simulink model "CubeX_LQR_2D"  (R2016b)
settings: Solver=FixedStepDiscrete  StartTime=0.0  StopTime=inf  FixedStep=Ts.base  RelTol=1e-3
PreLoadFcn:
  | waijung.modelPreload; % Required for working with Waijung Blockset. Do not remove.
InitFcn:
  | cubeparameters
  | LQR_2d
undefined symbols (not defined in the file): CPHA_1Edge, CPOL_Low, deg_, Duplex, FirstBit_MSB, Full, g, imu, K_lqr, Link, LQFP100, ST, STM32F407VG, STM32F4DISCOVERY, Ts
libraries: simulink x58, stm32f4_i2c_lib x12, stm32f4_io_lib x6, cube_lib x4, stm32f4_spi_lib x4, stm32f4_adc_lib x1, stm32f4_device_config_lib x1, BC_USB x1
(part 3 of 4)

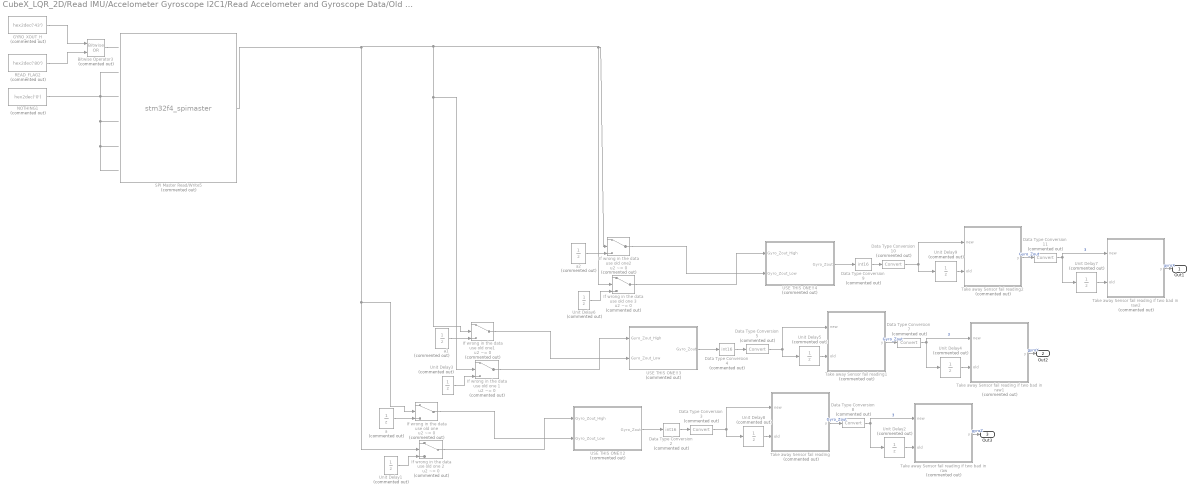
== system CubeX_LQR_2D/Read IMU/Accelometer Gyroscope I2C1/Read Accelometer and Gyroscope Data/Old gyro get data Used during SPI before ==
  " a" : UnitDelay  Commented=on  SampleTime=-1
  " a1" : UnitDelay  Commented=on  SampleTime=-1
  " a2" : UnitDelay  Commented=on  SampleTime=-1
  Bitwise Operator3 : simulink/Logic and Bit Operations/Bitwise Operator  Commented=on  logicop=OR  UseBitMask=off  NumInputPorts=2  BitMask=bin2dec('11011001')  BitMaskRealWorld=Stored Integer
  Data Type Conversion{3,5,7..8,10..11} (6 alike) : DataTypeConversion  Commented=on
  Data Type Conversion2 : DataTypeConversion  Commented=on  OutDataTypeStr=int16
  Data Type Conversion4 : DataTypeConversion  Commented=on  OutDataTypeStr=int16
  Data Type Conversion9 : DataTypeConversion  Commented=on  OutDataTypeStr=int16
  GYRO_XOUT_H : Constant  Commented=on  Value=hex2dec('43')  OutDataTypeStr=uint8
  If wrong in the data use old one : Switch  Commented=on  Criteria=u2 ~= 0
  If wrong in the data use old one 1 : Switch  Commented=on  Criteria=u2 ~= 0
  If wrong in the data use old one 2 : Switch  Commented=on  Criteria=u2 ~= 0
  If wrong in the data use old one 3 : Switch  Commented=on  Criteria=u2 ~= 0
  If wrong in the data use old one1 : Switch  Commented=on  Criteria=u2 ~= 0
  If wrong in the data use old one2 : Switch  Commented=on  Criteria=u2 ~= 0
  NOTHING1 : Constant  Commented=on  Value=hex2dec('0')  OutDataTypeStr=uint8
  READ_FLAG2 : Constant  Commented=on  Value=hex2dec('80')  OutDataTypeStr=uint8
  SPI Master Read/Write5 : S-Function  Commented=on  FunctionName=stm32f4_spimaster  Parameters=mode,configuration,module,datacount,inputtypearray,outputtypearray,confstr,sampletime,sampletimestr,blockid  SFunctionDeploymentMode=off  EnableBusSupport=off  mask(stm32f4_spimaster){configuration=Transaction, module=3, mode=Read/ Write, lastmodule=1, direction=Full-Duplex, dataformat=8bit/ FirstBit_MSB, prescaler=4, cpolcpha=CPOL_Low/ CPHA_1Edge, datacount='Could not find SPI Master Setup block for module 3', nssmode=Custom, nsspin=Not used, softnssport=E, softnsspin=0, sckpin=A5, misopin=A6, mosipin=A7, inputtypearray=[0], outputtypearray=[1 7], confstr=["SPI_Direction_2Lines_FullDuplex","8b","MSB","Low","1Edge","4","Soft","0","x","x","0","x","x","1","A","5","1","A","6","1","A","7","1","0","0","0","0","0","0","0","0","PP","0","UP"], sampletime=-1, sampletimestr=-1, blockid=AccelometerGyroscopeI2CReadAccelometerandGyroscopeDataOldgyrogetdataUsedduringSPIbeforeSPIMasterReadWrite5}
      mask prompts: module "SPI Module:"; lastmodule "Last module:"; dataformat "Data format:"; prescaler "Buad rate prescaler: Pclk/"; cpolcpha "Clock polarity (CPOL)/ Clock phase (CPHA):"; datacount "Data Read/Write count:"; nssmode "Slave/chip select (nSS, nCS) mode"; nsspin "Slave/chip select (nSS, nCS) pin"; softnssport "Slave/chip select port (nSS, nCS)"; softnsspin "Slave/chip select pin (nSS, nCS)"; sckpin "SCLK pin:"; misopin "MISO pin:"; mosipin "MOSI pin:"; inputtypearray "Input type array"; outputtypearray "Output type array"; confstr "Configuration string"; sampletime "Sample time (sec)"; sampletimestr "Compiled sample time (sec) in string"
      mask help:
      | Status:
      |  0 - Success.
      |  Otherwise - Fail.
      mask init:
      | stm32f4_spimaster_callback('init');
      mask Help: web(fullfile(waijungdocroot,'stm32f4_spimaster_readwrite.htm'), '-browser')
      mask TypeOptions configuration: Setup | Transaction
      mask Callback configuration: stm32f4_spimaster_callback('configuration');
      mask TypeOptions module: 1 | 2 | 3
      mask Callback module: stm32f4_spimaster_callback('module');
      mask TypeOptions mode: Read/ Write | Read | Write
      mask Callback mode: stm32f4_spimaster_callback('mode');
      mask TypeOptions direction: Full-Duplex | Half-Duplex_Tx | Half-Duplex_Rx
      mask Callback direction: stm32f4_spimaster_callback('direction');
      mask TypeOptions dataformat: 8bit/ FirstBit_MSB | 8bit/ FirstBit_LSB | 16bit/ FirstBit_MSB | 16bit/ FirstBit_LSB
      mask TypeOptions prescaler: 2 | 4 | 8 | 16 | 32 | 64 | 128 | 256
      mask TypeOptions cpolcpha: CPOL_Low/ CPHA_1Edge | CPOL_Low/ CPHA_2Edge | CPOL_High/ CPHA_1Edge | CPOL_High/ CPHA_2Edge
      mask Callback datacount: stm32f4_spimaster_callback('datacount');
      mask TypeOptions nssmode: Hardware | Software | Custom
      mask Callback nssmode: stm32f4_spimaster_callback('nssmode');
      mask TypeOptions nsspin: Not used | A4 | A15
      mask TypeOptions softnssport: A | B | C | D | E | F | G | H | I
      mask TypeOptions softnsspin: 0 | 1 | 2 | 3 | 4 | 5 | 6 | 7 | 8 | 9 | 10 | 11 | 12 | 13 | 14 | 15
      mask TypeOptions sckpin: Not used | A5 | B3
      mask TypeOptions misopin: Not used | A6 | B4
      mask TypeOptions mosipin: Not used | A7 | B5
      mask Callback confstr: stm32f4_spimaster_callback('confstr');
      mask Callback sampletime: stm32f4_spimaster_callback('sampletime');
      mask Callback sampletimestr: stm32f4_spimaster_callback('sampletimestr');
      mask Callback blockid: stm32f4_spimaster_callback('blockid');
      mask Display: text(0.5, 0.5, 'Module: SPI3 (Master)\nRead/ Write\nTs (sec): -1','ver','middle','hor','center');port_label('output', 1,'Status');
  Take away Sensor fail reading : MATLAB Function  Commented=on  TreatAsAtomicUnit=on
  Take away Sensor fail reading if two bad in raw : MATLAB Function  Commented=on  TreatAsAtomicUnit=on
  Take away Sensor fail reading if two bad in raw1 : MATLAB Function  Commented=on  TreatAsAtomicUnit=on
  Take away Sensor fail reading if two bad in raw2 : MATLAB Function  Commented=on  TreatAsAtomicUnit=on
  Take away Sensor fail reading1 : MATLAB Function  Commented=on  TreatAsAtomicUnit=on
  Take away Sensor fail reading2 : MATLAB Function  Commented=on  TreatAsAtomicUnit=on
  USE THIS ONE!!2 : Subsystem  Commented=on
  USE THIS ONE!!3 : Subsystem  Commented=on
  USE THIS ONE!!4 : Subsystem  Commented=on
  Unit Delay1 : UnitDelay  Commented=on  SampleTime=-1
  Unit Delay{2,4..5,7..9} (6 alike) : UnitDelay  Commented=on  InitialCondition=-40.45  SampleTime=-1
  Unit Delay3 : UnitDelay  Commented=on  SampleTime=-1
  Unit Delay6 : UnitDelay  Commented=on  SampleTime=-1
  Out1 : Outport
  Out2 : Outport  Port=2
  Out3 : Outport  Port=3
  wires:
  Data Type Conversion8/1 -> Unit Delay2/1, Take away Sensor fail reading if two bad in raw/1(new)  "3"
  Bitwise Operator3/1 -> ?
  USE THIS ONE!!2/1(Gyro_Zout) -> Data Type Conversion2/1
  GYRO_XOUT_H/1 -> Bitwise Operator3/1
  Unit Delay8/1 -> Take away Sensor fail reading/2(old)
  ? -> If wrong in the data use old one 2/1, Unit Delay1/1
  READ_FLAG2/1 -> Bitwise Operator3/2
  If wrong in the data use old one 2/1 -> USE THIS ONE!!2/1("Gyro_Zout_High ")
  If wrong in the data use old one/1 -> USE THIS ONE!!2/2(Gyro_Zout_Low)
  ? -> " a"/1, If wrong in the data use old one/1  "Gyro_zou_Lowt"
  " a"/1 -> If wrong in the data use old one/3
  Data Type Conversion2/1 -> Data Type Conversion3/1
  NOTHING1/1 -> ?
  Unit Delay1/1 -> If wrong in the data use old one 2/3
  Take away Sensor fail reading/1(y) -> Data Type Conversion8/1  "Gyro_Zout"
  Unit Delay2/1 -> Take away Sensor fail reading if two bad in raw/2(old)
  Unit Delay7/1 -> Take away Sensor fail reading if two bad in raw2/2(old)
  If wrong in the data use old one1/1 -> USE THIS ONE!!3/2(Gyro_Zout_Low)
  ? -> Unit Delay3/1, If wrong in the data use old one 1/1  "Gyro_zou_Lowt"
  " a2"/1 -> If wrong in the data use old one2/3
  Take away Sensor fail reading2/1(y) -> Data Type Conversion11/1  "Gyro_Zout"
  Data Type Conversion10/1 -> Take away Sensor fail reading2/1(new), Unit Delay9/1
  Data Type Conversion11/1 -> Unit Delay7/1, Take away Sensor fail reading if two bad in raw2/1(new)  "3"
  Unit Delay5/1 -> Take away Sensor fail reading1/2(old)
  SPI Master Read/Write5/1 -> If wrong in the data use old one2/2, If wrong in the data use old one 3/2, If wrong in the data use old one 1/2, If wrong in the data use old one1/2, If wrong in the data use old one 2/2, If wrong in the data use old one/2
  ? -> " a2"/1, If wrong in the data use old one2/1  "Gyro_zou_Lowt"
  ? -> " a1"/1, If wrong in the data use old one1/1  "Gyro_zou_Lowt"
  Data Type Conversion7/1 -> Unit Delay4/1, Take away Sensor fail reading if two bad in raw1/1(new)  "3"
  Data Type Conversion3/1 -> Take away Sensor fail reading/1(new), Unit Delay8/1
  Data Type Conversion4/1 -> Data Type Conversion5/1
  Data Type Conversion9/1 -> Data Type Conversion10/1
  USE THIS ONE!!3/1(Gyro_Zout) -> Data Type Conversion4/1
  " a1"/1 -> If wrong in the data use old one1/3
  Unit Delay6/1 -> If wrong in the data use old one 3/3
  USE THIS ONE!!4/1(Gyro_Zout) -> Data Type Conversion9/1
  If wrong in the data use old one 1/1 -> USE THIS ONE!!3/1("Gyro_Zout_High ")
  If wrong in the data use old one2/1 -> USE THIS ONE!!4/2(Gyro_Zout_Low)
  Unit Delay3/1 -> If wrong in the data use old one 1/3
  Data Type Conversion5/1 -> Take away Sensor fail reading1/1(new), Unit Delay5/1
  ? -> If wrong in the data use old one 3/1, Unit Delay6/1  "Gyro_zou_Lowt"
  If wrong in the data use old one 3/1 -> USE THIS ONE!!4/1("Gyro_Zout_High ")
  Unit Delay9/1 -> Take away Sensor fail reading2/2(old)
  Unit Delay4/1 -> Take away Sensor fail reading if two bad in raw1/2(old)
  Take away Sensor fail reading1/1(y) -> Data Type Conversion7/1  "Gyro_Zout"
  Take away Sensor fail reading if two bad in raw2/1(y) -> Out1/1  "gyroX"
  Take away Sensor fail reading if two bad in raw/1(y) -> Out3/1  "gyroZ"
  Take away Sensor fail reading if two bad in raw1/1(y) -> Out2/1  "gyroY"

== system CubeX_LQR_2D/Read IMU/Accelometer Gyroscope I2C1/Read Accelometer and Gyroscope Data/Turn the MSB and LSB into a signed 16-bit integer AccX ==
  note: Bitshift up the MSB bits and bitwise OR the LSB
      | into a int16
  MSB : Inport
  LSB : Inport  Port=2
  Bitwise Operator2 : simulink/Logic and Bit Operations/Bitwise Operator  logicop=OR  UseBitMask=off  NumInputPorts=2  BitMask=bin2dec('11011001')  BitMaskRealWorld=Stored Integer
  Data Type Conversion6 : DataTypeConversion  OutDataTypeStr=uint16
  Data Type Conversion7 : DataTypeConversion  OutDataTypeStr=uint16
  Shift Arithmetic2 : ArithShift  BitShiftNumber=-8
  out16b : Outport
  wires:
  LSB/1 -> Data Type Conversion6/1
  Bitwise Operator2/1 -> out16b/1
  MSB/1 -> Data Type Conversion7/1
  Data Type Conversion7/1 -> Shift Arithmetic2/1
  Data Type Conversion6/1 -> Bitwise Operator2/2
  Shift Arithmetic2/1 -> Bitwise Operator2/1

== system CubeX_LQR_2D/Read IMU/Accelometer Gyroscope I2C1/Read Accelometer and Gyroscope Data/Turn the MSB and LSB into a signed 16-bit integer AccY ==
  note: Bitshift up the MSB bits and bitwise OR the LSB
      | into a int16
  MSB : Inport
  LSB : Inport  Port=2
  Bitwise Operator2 : simulink/Logic and Bit Operations/Bitwise Operator  logicop=OR  UseBitMask=off  NumInputPorts=2  BitMask=bin2dec('11011001')  BitMaskRealWorld=Stored Integer
  Data Type Conversion6 : DataTypeConversion  OutDataTypeStr=uint16
  Data Type Conversion7 : DataTypeConversion  OutDataTypeStr=uint16
  Shift Arithmetic2 : ArithShift  BitShiftNumber=-8
  out16b : Outport
  wires:
  LSB/1 -> Data Type Conversion6/1
  Bitwise Operator2/1 -> out16b/1
  MSB/1 -> Data Type Conversion7/1
  Data Type Conversion7/1 -> Shift Arithmetic2/1
  Data Type Conversion6/1 -> Bitwise Operator2/2
  Shift Arithmetic2/1 -> Bitwise Operator2/1

== system CubeX_LQR_2D/Read IMU/Accelometer Gyroscope I2C1/Read Accelometer and Gyroscope Data/Turn the MSB and LSB into a signed 16-bit integer AccZ ==
  note: Bitshift up the MSB bits and bitwise OR the LSB
      | into a int16
  MSB : Inport
  LSB : Inport  Port=2
  Bitwise Operator2 : simulink/Logic and Bit Operations/Bitwise Operator  logicop=OR  UseBitMask=off  NumInputPorts=2  BitMask=bin2dec('11011001')  BitMaskRealWorld=Stored Integer
  Data Type Conversion6 : DataTypeConversion  OutDataTypeStr=uint16
  Data Type Conversion7 : DataTypeConversion  OutDataTypeStr=uint16
  Shift Arithmetic2 : ArithShift  BitShiftNumber=-8
  out16b : Outport
  wires:
  LSB/1 -> Data Type Conversion6/1
  Bitwise Operator2/1 -> out16b/1
  MSB/1 -> Data Type Conversion7/1
  Data Type Conversion7/1 -> Shift Arithmetic2/1
  Data Type Conversion6/1 -> Bitwise Operator2/2
  Shift Arithmetic2/1 -> Bitwise Operator2/1

== system CubeX_LQR_2D/Read IMU/Accelometer Gyroscope I2C1/Read Accelometer and Gyroscope Data/Turn the MSB and LSB into a signed 16-bit integer GyroX ==
  note: Bitshift up the MSB bits and bitwise OR the LSB
      | into a int16
  MSB : Inport
  LSB : Inport  Port=2
  Bitwise Operator2 : simulink/Logic and Bit Operations/Bitwise Operator  logicop=OR  UseBitMask=off  NumInputPorts=2  BitMask=bin2dec('11011001')  BitMaskRealWorld=Stored Integer
  Data Type Conversion6 : DataTypeConversion  OutDataTypeStr=uint16
  Data Type Conversion7 : DataTypeConversion  OutDataTypeStr=uint16
  Shift Arithmetic2 : ArithShift  BitShiftNumber=-8
  out16b : Outport
  wires:
  LSB/1 -> Data Type Conversion6/1
  Bitwise Operator2/1 -> out16b/1
  MSB/1 -> Data Type Conversion7/1
  Data Type Conversion7/1 -> Shift Arithmetic2/1
  Data Type Conversion6/1 -> Bitwise Operator2/2
  Shift Arithmetic2/1 -> Bitwise Operator2/1

== system CubeX_LQR_2D/Read IMU/Accelometer Gyroscope I2C1/Read Accelometer and Gyroscope Data/Turn the MSB and LSB into a signed 16-bit integer GyroY ==
  note: Bitshift up the MSB bits and bitwise OR the LSB
      | into a int16
  MSB : Inport
  LSB : Inport  Port=2
  Bitwise Operator2 : simulink/Logic and Bit Operations/Bitwise Operator  logicop=OR  UseBitMask=off  NumInputPorts=2  BitMask=bin2dec('11011001')  BitMaskRealWorld=Stored Integer
  Data Type Conversion6 : DataTypeConversion  OutDataTypeStr=uint16
  Data Type Conversion7 : DataTypeConversion  OutDataTypeStr=uint16
  Shift Arithmetic2 : ArithShift  BitShiftNumber=-8
  out16b : Outport
  wires:
  LSB/1 -> Data Type Conversion6/1
  Bitwise Operator2/1 -> out16b/1
  MSB/1 -> Data Type Conversion7/1
  Data Type Conversion7/1 -> Shift Arithmetic2/1
  Data Type Conversion6/1 -> Bitwise Operator2/2
  Shift Arithmetic2/1 -> Bitwise Operator2/1

== system CubeX_LQR_2D/Read IMU/Accelometer Gyroscope I2C1/Read Accelometer and Gyroscope Data/Turn the MSB and LSB into a signed 16-bit integer GyroZ ==
  note: Bitshift up the MSB bits and bitwise OR the LSB
      | into a int16
  MSB : Inport
  LSB : Inport  Port=2
  Bitwise Operator2 : simulink/Logic and Bit Operations/Bitwise Operator  logicop=OR  UseBitMask=off  NumInputPorts=2  BitMask=bin2dec('11011001')  BitMaskRealWorld=Stored Integer
  Data Type Conversion6 : DataTypeConversion  OutDataTypeStr=uint16
  Data Type Conversion7 : DataTypeConversion  OutDataTypeStr=uint16
  Shift Arithmetic2 : ArithShift  BitShiftNumber=-8
  out16b : Outport
  wires:
  LSB/1 -> Data Type Conversion6/1
  Bitwise Operator2/1 -> out16b/1
  MSB/1 -> Data Type Conversion7/1
  Data Type Conversion7/1 -> Shift Arithmetic2/1
  Data Type Conversion6/1 -> Bitwise Operator2/2
  Shift Arithmetic2/1 -> Bitwise Operator2/1

== system CubeX_LQR_2D/Read IMU/Accelometer Gyroscope I2C3/MPU9250 Init/Write Configuration ==
  note: Enable BYPSS_EN in INT_PIN_CFG register to be able to read magnetometer trough I2C
  SlvAddr : Inport
  Enable : EnablePort
  BYPASS_EN : Constant  Value=hex2dec('02')  OutDataTypeStr=uint8  SampleTime=-1
  I2C Master Read/Write1 : stm32f4_i2c_lib/I2C Master Read//Write  configuration=Transaction  module=3  lastmodule=3  transfer=Blocking  dutycycle=TLow/THigh = 2  clkspeed=400  timeout=25  writecount=2  readcount=0  sdapin=C9  sclpin=A8  waitwritetime=0  forcestop=off  inputtypearray=[3 3 3 3]  outputtypearray=[1 3]  confstr="[\"C\",\"9\",\"A\",\"8\",\"1\",\"3\",\"4\",\"2\",\"I2C_DutyCycle_2\",\"0\",\"off\"]"  sampletime=-1  sampletimestr=0.008  blockid=ReadIMUAccelometerGyroscopeI2C3MPU9250InitWriteConfigurationI2CMasterReadWrite1
  INT_PIN_CFG1 : Constant  Value=hex2dec('37')  OutDataTypeStr=uint8  SampleTime=-1
  Terminator : Terminator
  wires:
  I2C Master Read/Write1/1 -> Terminator/1
  BYPASS_EN/1 -> I2C Master Read/Write1/3
  INT_PIN_CFG1/1 -> I2C Master Read/Write1/2
  SlvAddr/1 -> I2C Master Read/Write1/1

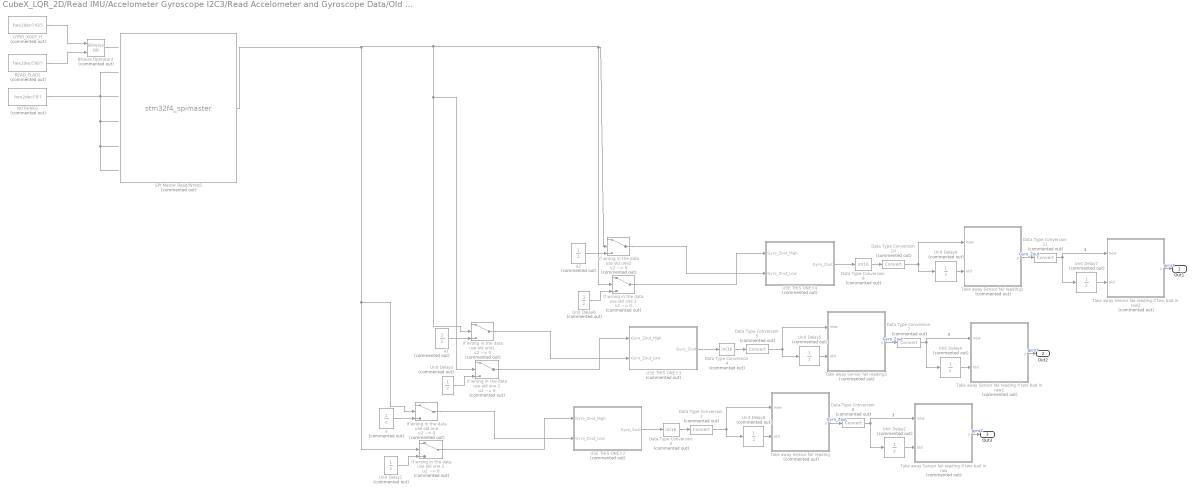
== system CubeX_LQR_2D/Read IMU/Accelometer Gyroscope I2C3/Read Accelometer and Gyroscope Data/Old gyro get data Used during SPI before ==
  " a" : UnitDelay  Commented=on  SampleTime=-1
  " a1" : UnitDelay  Commented=on  SampleTime=-1
  " a2" : UnitDelay  Commented=on  SampleTime=-1
  Bitwise Operator3 : simulink/Logic and Bit Operations/Bitwise Operator  Commented=on  logicop=OR  UseBitMask=off  NumInputPorts=2  BitMask=bin2dec('11011001')  BitMaskRealWorld=Stored Integer
  Data Type Conversion{3,5,7..8,10..11} (6 alike) : DataTypeConversion  Commented=on
  Data Type Conversion2 : DataTypeConversion  Commented=on  OutDataTypeStr=int16
  Data Type Conversion4 : DataTypeConversion  Commented=on  OutDataTypeStr=int16
  Data Type Conversion9 : DataTypeConversion  Commented=on  OutDataTypeStr=int16
  GYRO_XOUT_H : Constant  Commented=on  Value=hex2dec('43')  OutDataTypeStr=uint8
  If wrong in the data use old one : Switch  Commented=on  Criteria=u2 ~= 0
  If wrong in the data use old one 1 : Switch  Commented=on  Criteria=u2 ~= 0
  If wrong in the data use old one 2 : Switch  Commented=on  Criteria=u2 ~= 0
  If wrong in the data use old one 3 : Switch  Commented=on  Criteria=u2 ~= 0
  If wrong in the data use old one1 : Switch  Commented=on  Criteria=u2 ~= 0
  If wrong in the data use old one2 : Switch  Commented=on  Criteria=u2 ~= 0
  NOTHING1 : Constant  Commented=on  Value=hex2dec('0')  OutDataTypeStr=uint8
  READ_FLAG2 : Constant  Commented=on  Value=hex2dec('80')  OutDataTypeStr=uint8
  SPI Master Read/Write5 : S-Function  Commented=on  FunctionName=stm32f4_spimaster  Parameters=mode,configuration,module,datacount,inputtypearray,outputtypearray,confstr,sampletime,sampletimestr,blockid  SFunctionDeploymentMode=off  EnableBusSupport=off  mask(stm32f4_spimaster){configuration=Transaction, module=3, mode=Read/ Write, lastmodule=1, direction=Full-Duplex, dataformat=8bit/ FirstBit_MSB, prescaler=4, cpolcpha=CPOL_Low/ CPHA_1Edge, datacount='Could not find SPI Master Setup block for module 3', nssmode=Custom, nsspin=Not used, softnssport=E, softnsspin=0, sckpin=A5, misopin=A6, mosipin=A7, inputtypearray=[0], outputtypearray=[1 7], confstr=["SPI_Direction_2Lines_FullDuplex","8b","MSB","Low","1Edge","4","Soft","0","x","x","0","x","x","1","A","5","1","A","6","1","A","7","1","0","0","0","0","0","0","0","0","PP","0","UP"], sampletime=-1, sampletimestr=-1, blockid=AccelometerGyroscopeI2CReadAccelometerandGyroscopeDataOldgyrogetdataUsedduringSPIbeforeSPIMasterReadWrite5}
      mask prompts: module "SPI Module:"; lastmodule "Last module:"; dataformat "Data format:"; prescaler "Buad rate prescaler: Pclk/"; cpolcpha "Clock polarity (CPOL)/ Clock phase (CPHA):"; datacount "Data Read/Write count:"; nssmode "Slave/chip select (nSS, nCS) mode"; nsspin "Slave/chip select (nSS, nCS) pin"; softnssport "Slave/chip select port (nSS, nCS)"; softnsspin "Slave/chip select pin (nSS, nCS)"; sckpin "SCLK pin:"; misopin "MISO pin:"; mosipin "MOSI pin:"; inputtypearray "Input type array"; outputtypearray "Output type array"; confstr "Configuration string"; sampletime "Sample time (sec)"; sampletimestr "Compiled sample time (sec) in string"
      mask help:
      | Status:
      |  0 - Success.
      |  Otherwise - Fail.
      mask init:
      | stm32f4_spimaster_callback('init');
      mask Help: web(fullfile(waijungdocroot,'stm32f4_spimaster_readwrite.htm'), '-browser')
      mask TypeOptions configuration: Setup | Transaction
      mask Callback configuration: stm32f4_spimaster_callback('configuration');
      mask TypeOptions module: 1 | 2 | 3
      mask Callback module: stm32f4_spimaster_callback('module');
      mask TypeOptions mode: Read/ Write | Read | Write
      mask Callback mode: stm32f4_spimaster_callback('mode');
      mask TypeOptions direction: Full-Duplex | Half-Duplex_Tx | Half-Duplex_Rx
      mask Callback direction: stm32f4_spimaster_callback('direction');
      mask TypeOptions dataformat: 8bit/ FirstBit_MSB | 8bit/ FirstBit_LSB | 16bit/ FirstBit_MSB | 16bit/ FirstBit_LSB
      mask TypeOptions prescaler: 2 | 4 | 8 | 16 | 32 | 64 | 128 | 256
      mask TypeOptions cpolcpha: CPOL_Low/ CPHA_1Edge | CPOL_Low/ CPHA_2Edge | CPOL_High/ CPHA_1Edge | CPOL_High/ CPHA_2Edge
      mask Callback datacount: stm32f4_spimaster_callback('datacount');
      mask TypeOptions nssmode: Hardware | Software | Custom
      mask Callback nssmode: stm32f4_spimaster_callback('nssmode');
      mask TypeOptions nsspin: Not used | A4 | A15
      mask TypeOptions softnssport: A | B | C | D | E | F | G | H | I
      mask TypeOptions softnsspin: 0 | 1 | 2 | 3 | 4 | 5 | 6 | 7 | 8 | 9 | 10 | 11 | 12 | 13 | 14 | 15
      mask TypeOptions sckpin: Not used | A5 | B3
      mask TypeOptions misopin: Not used | A6 | B4
      mask TypeOptions mosipin: Not used | A7 | B5
      mask Callback confstr: stm32f4_spimaster_callback('confstr');
      mask Callback sampletime: stm32f4_spimaster_callback('sampletime');
      mask Callback sampletimestr: stm32f4_spimaster_callback('sampletimestr');
      mask Callback blockid: stm32f4_spimaster_callback('blockid');
      mask Display: text(0.5, 0.5, 'Module: SPI3 (Master)\nRead/ Write\nTs (sec): -1','ver','middle','hor','center');port_label('output', 1,'Status');
  Take away Sensor fail reading : MATLAB Function  Commented=on  TreatAsAtomicUnit=on
  Take away Sensor fail reading if two bad in raw : MATLAB Function  Commented=on  TreatAsAtomicUnit=on
  Take away Sensor fail reading if two bad in raw1 : MATLAB Function  Commented=on  TreatAsAtomicUnit=on
  Take away Sensor fail reading if two bad in raw2 : MATLAB Function  Commented=on  TreatAsAtomicUnit=on
  Take away Sensor fail reading1 : MATLAB Function  Commented=on  TreatAsAtomicUnit=on
  Take away Sensor fail reading2 : MATLAB Function  Commented=on  TreatAsAtomicUnit=on
  USE THIS ONE!!2 : Subsystem  Commented=on
  USE THIS ONE!!3 : Subsystem  Commented=on
  USE THIS ONE!!4 : Subsystem  Commented=on
  Unit Delay1 : UnitDelay  Commented=on  SampleTime=-1
  Unit Delay{2,4..5,7..9} (6 alike) : UnitDelay  Commented=on  InitialCondition=-40.45  SampleTime=-1
  Unit Delay3 : UnitDelay  Commented=on  SampleTime=-1
  Unit Delay6 : UnitDelay  Commented=on  SampleTime=-1
  Out1 : Outport
  Out2 : Outport  Port=2
  Out3 : Outport  Port=3
  wires:
  Data Type Conversion8/1 -> Unit Delay2/1, Take away Sensor fail reading if two bad in raw/1(new)  "3"
  Bitwise Operator3/1 -> ?
  USE THIS ONE!!2/1(Gyro_Zout) -> Data Type Conversion2/1
  GYRO_XOUT_H/1 -> Bitwise Operator3/1
  Unit Delay8/1 -> Take away Sensor fail reading/2(old)
  ? -> If wrong in the data use old one 2/1, Unit Delay1/1
  READ_FLAG2/1 -> Bitwise Operator3/2
  If wrong in the data use old one 2/1 -> USE THIS ONE!!2/1("Gyro_Zout_High ")
  If wrong in the data use old one/1 -> USE THIS ONE!!2/2(Gyro_Zout_Low)
  ? -> " a"/1, If wrong in the data use old one/1  "Gyro_zou_Lowt"
  " a"/1 -> If wrong in the data use old one/3
  Data Type Conversion2/1 -> Data Type Conversion3/1
  NOTHING1/1 -> ?
  Unit Delay1/1 -> If wrong in the data use old one 2/3
  Take away Sensor fail reading/1(y) -> Data Type Conversion8/1  "Gyro_Zout"
  Unit Delay2/1 -> Take away Sensor fail reading if two bad in raw/2(old)
  Unit Delay7/1 -> Take away Sensor fail reading if two bad in raw2/2(old)
  If wrong in the data use old one1/1 -> USE THIS ONE!!3/2(Gyro_Zout_Low)
  ? -> Unit Delay3/1, If wrong in the data use old one 1/1  "Gyro_zou_Lowt"
  " a2"/1 -> If wrong in the data use old one2/3
  Take away Sensor fail reading2/1(y) -> Data Type Conversion11/1  "Gyro_Zout"
  Data Type Conversion10/1 -> Take away Sensor fail reading2/1(new), Unit Delay9/1
  Data Type Conversion11/1 -> Unit Delay7/1, Take away Sensor fail reading if two bad in raw2/1(new)  "3"
  Unit Delay5/1 -> Take away Sensor fail reading1/2(old)
  SPI Master Read/Write5/1 -> If wrong in the data use old one2/2, If wrong in the data use old one 3/2, If wrong in the data use old one 1/2, If wrong in the data use old one1/2, If wrong in the data use old one 2/2, If wrong in the data use old one/2
  ? -> " a2"/1, If wrong in the data use old one2/1  "Gyro_zou_Lowt"
  ? -> " a1"/1, If wrong in the data use old one1/1  "Gyro_zou_Lowt"
  Data Type Conversion7/1 -> Unit Delay4/1, Take away Sensor fail reading if two bad in raw1/1(new)  "3"
  Data Type Conversion3/1 -> Take away Sensor fail reading/1(new), Unit Delay8/1
  Data Type Conversion4/1 -> Data Type Conversion5/1
  Data Type Conversion9/1 -> Data Type Conversion10/1
  USE THIS ONE!!3/1(Gyro_Zout) -> Data Type Conversion4/1
  " a1"/1 -> If wrong in the data use old one1/3
  Unit Delay6/1 -> If wrong in the data use old one 3/3
  USE THIS ONE!!4/1(Gyro_Zout) -> Data Type Conversion9/1
  If wrong in the data use old one 1/1 -> USE THIS ONE!!3/1("Gyro_Zout_High ")
  If wrong in the data use old one2/1 -> USE THIS ONE!!4/2(Gyro_Zout_Low)
  Unit Delay3/1 -> If wrong in the data use old one 1/3
  Data Type Conversion5/1 -> Take away Sensor fail reading1/1(new), Unit Delay5/1
  ? -> If wrong in the data use old one 3/1, Unit Delay6/1  "Gyro_zou_Lowt"
  If wrong in the data use old one 3/1 -> USE THIS ONE!!4/1("Gyro_Zout_High ")
  Unit Delay9/1 -> Take away Sensor fail reading2/2(old)
  Unit Delay4/1 -> Take away Sensor fail reading if two bad in raw1/2(old)
  Take away Sensor fail reading1/1(y) -> Data Type Conversion7/1  "Gyro_Zout"
  Take away Sensor fail reading if two bad in raw2/1(y) -> Out1/1  "gyroX"
  Take away Sensor fail reading if two bad in raw/1(y) -> Out3/1  "gyroZ"
  Take away Sensor fail reading if two bad in raw1/1(y) -> Out2/1  "gyroY"

== system CubeX_LQR_2D/Read IMU/Accelometer Gyroscope I2C3/Read Accelometer and Gyroscope Data/Turn the MSB and LSB into a signed 16-bit integer AccX ==
  note: Bitshift up the MSB bits and bitwise OR the LSB
      | into a int16
  MSB : Inport
  LSB : Inport  Port=2
  Bitwise Operator2 : simulink/Logic and Bit Operations/Bitwise Operator  logicop=OR  UseBitMask=off  NumInputPorts=2  BitMask=bin2dec('11011001')  BitMaskRealWorld=Stored Integer
  Data Type Conversion6 : DataTypeConversion  OutDataTypeStr=uint16
  Data Type Conversion7 : DataTypeConversion  OutDataTypeStr=uint16
  Shift Arithmetic2 : ArithShift  BitShiftNumber=-8
  out16b : Outport
  wires:
  LSB/1 -> Data Type Conversion6/1
  Bitwise Operator2/1 -> out16b/1
  MSB/1 -> Data Type Conversion7/1
  Data Type Conversion7/1 -> Shift Arithmetic2/1
  Data Type Conversion6/1 -> Bitwise Operator2/2
  Shift Arithmetic2/1 -> Bitwise Operator2/1

== system CubeX_LQR_2D/Read IMU/Accelometer Gyroscope I2C3/Read Accelometer and Gyroscope Data/Turn the MSB and LSB into a signed 16-bit integer AccY ==
  note: Bitshift up the MSB bits and bitwise OR the LSB
      | into a int16
  MSB : Inport
  LSB : Inport  Port=2
  Bitwise Operator2 : simulink/Logic and Bit Operations/Bitwise Operator  logicop=OR  UseBitMask=off  NumInputPorts=2  BitMask=bin2dec('11011001')  BitMaskRealWorld=Stored Integer
  Data Type Conversion6 : DataTypeConversion  OutDataTypeStr=uint16
  Data Type Conversion7 : DataTypeConversion  OutDataTypeStr=uint16
  Shift Arithmetic2 : ArithShift  BitShiftNumber=-8
  out16b : Outport
  wires:
  LSB/1 -> Data Type Conversion6/1
  Bitwise Operator2/1 -> out16b/1
  MSB/1 -> Data Type Conversion7/1
  Data Type Conversion7/1 -> Shift Arithmetic2/1
  Data Type Conversion6/1 -> Bitwise Operator2/2
  Shift Arithmetic2/1 -> Bitwise Operator2/1

== system CubeX_LQR_2D/Read IMU/Accelometer Gyroscope I2C3/Read Accelometer and Gyroscope Data/Turn the MSB and LSB into a signed 16-bit integer AccZ ==
  note: Bitshift up the MSB bits and bitwise OR the LSB
      | into a int16
  MSB : Inport
  LSB : Inport  Port=2
  Bitwise Operator2 : simulink/Logic and Bit Operations/Bitwise Operator  logicop=OR  UseBitMask=off  NumInputPorts=2  BitMask=bin2dec('11011001')  BitMaskRealWorld=Stored Integer
  Data Type Conversion6 : DataTypeConversion  OutDataTypeStr=uint16
  Data Type Conversion7 : DataTypeConversion  OutDataTypeStr=uint16
  Shift Arithmetic2 : ArithShift  BitShiftNumber=-8
  out16b : Outport
  wires:
  LSB/1 -> Data Type Conversion6/1
  Bitwise Operator2/1 -> out16b/1
  MSB/1 -> Data Type Conversion7/1
  Data Type Conversion7/1 -> Shift Arithmetic2/1
  Data Type Conversion6/1 -> Bitwise Operator2/2
  Shift Arithmetic2/1 -> Bitwise Operator2/1

== system CubeX_LQR_2D/Read IMU/Accelometer Gyroscope I2C3/Read Accelometer and Gyroscope Data/Turn the MSB and LSB into a signed 16-bit integer GyroX ==
  note: Bitshift up the MSB bits and bitwise OR the LSB
      | into a int16
  MSB : Inport
  LSB : Inport  Port=2
  Bitwise Operator2 : simulink/Logic and Bit Operations/Bitwise Operator  logicop=OR  UseBitMask=off  NumInputPorts=2  BitMask=bin2dec('11011001')  BitMaskRealWorld=Stored Integer
  Data Type Conversion6 : DataTypeConversion  OutDataTypeStr=uint16
  Data Type Conversion7 : DataTypeConversion  OutDataTypeStr=uint16
  Shift Arithmetic2 : ArithShift  BitShiftNumber=-8
  out16b : Outport
  wires:
  LSB/1 -> Data Type Conversion6/1
  Bitwise Operator2/1 -> out16b/1
  MSB/1 -> Data Type Conversion7/1
  Data Type Conversion7/1 -> Shift Arithmetic2/1
  Data Type Conversion6/1 -> Bitwise Operator2/2
  Shift Arithmetic2/1 -> Bitwise Operator2/1

== system CubeX_LQR_2D/Read IMU/Accelometer Gyroscope I2C3/Read Accelometer and Gyroscope Data/Turn the MSB and LSB into a signed 16-bit integer GyroY ==
  note: Bitshift up the MSB bits and bitwise OR the LSB
      | into a int16
  MSB : Inport
  LSB : Inport  Port=2
  Bitwise Operator2 : simulink/Logic and Bit Operations/Bitwise Operator  logicop=OR  UseBitMask=off  NumInputPorts=2  BitMask=bin2dec('11011001')  BitMaskRealWorld=Stored Integer
  Data Type Conversion6 : DataTypeConversion  OutDataTypeStr=uint16
  Data Type Conversion7 : DataTypeConversion  OutDataTypeStr=uint16
  Shift Arithmetic2 : ArithShift  BitShiftNumber=-8
  out16b : Outport
  wires:
  LSB/1 -> Data Type Conversion6/1
  Bitwise Operator2/1 -> out16b/1
  MSB/1 -> Data Type Conversion7/1
  Data Type Conversion7/1 -> Shift Arithmetic2/1
  Data Type Conversion6/1 -> Bitwise Operator2/2
  Shift Arithmetic2/1 -> Bitwise Operator2/1

== system CubeX_LQR_2D/Read IMU/Accelometer Gyroscope I2C3/Read Accelometer and Gyroscope Data/Turn the MSB and LSB into a signed 16-bit integer GyroZ ==
  note: Bitshift up the MSB bits and bitwise OR the LSB
      | into a int16
  MSB : Inport
  LSB : Inport  Port=2
  Bitwise Operator2 : simulink/Logic and Bit Operations/Bitwise Operator  logicop=OR  UseBitMask=off  NumInputPorts=2  BitMask=bin2dec('11011001')  BitMaskRealWorld=Stored Integer
  Data Type Conversion6 : DataTypeConversion  OutDataTypeStr=uint16
  Data Type Conversion7 : DataTypeConversion  OutDataTypeStr=uint16
  Shift Arithmetic2 : ArithShift  BitShiftNumber=-8
  out16b : Outport
  wires:
  LSB/1 -> Data Type Conversion6/1
  Bitwise Operator2/1 -> out16b/1
  MSB/1 -> Data Type Conversion7/1
  Data Type Conversion7/1 -> Shift Arithmetic2/1
  Data Type Conversion6/1 -> Bitwise Operator2/2
  Shift Arithmetic2/1 -> Bitwise Operator2/1

== system CubeX_LQR_2D/Read IMU/Magnetometer I2C1/AK8963 Init /Write Configuration ==
  SlvAddr : Inport
  RegAddr : Inport  Port=2
  Enable : EnablePort
  I2C Master Read/Write1 : stm32f4_i2c_lib/I2C Master Read//Write  configuration=Transaction  module=1  lastmodule=3  transfer=Blocking  dutycycle=TLow/THigh = 2  clkspeed=400  timeout=25  writecount=2  readcount=0  sdapin=C9  sclpin=A8  waitwritetime=0  forcestop=off  inputtypearray=[3 3 3 3]  outputtypearray=[1 3]  confstr="[\"C\",\"9\",\"A\",\"8\",\"1\",\"1\",\"6\",\"0\",\"I2C_DutyCycle_2\",\"0\",\"off\"]"  sampletime=-1  sampletimestr=0.002  blockid=ReadIMUMagnetometerI2CAK8963InitWriteConfigurationI2CMasterReadWrite1
  Terminator : Terminator
  "bit[5] : 16-bit output bit[3:0] - Continuous measurement mode 2" : Constant  Value=hex2dec('16')  OutDataTypeStr=uint8  SampleTime=-1
  wires:
  RegAddr/1 -> I2C Master Read/Write1/2
  SlvAddr/1 -> I2C Master Read/Write1/1
  I2C Master Read/Write1/1 -> Terminator/1
  "bit[5] : 16-bit output bit[3:0] - Continuous measurement mode 2"/1 -> I2C Master Read/Write1/3

== system CubeX_LQR_2D/Read IMU/Magnetometer I2C1/Read Magnetometer Data/Turn the MSB and LSB into a signed 16-bit integer MagX ==
  low : Inport
  high : Inport  Port=2
  Bitwise Operator2 : simulink/Logic and Bit Operations/Bitwise Operator  logicop=OR  UseBitMask=off  NumInputPorts=2  BitMask=bin2dec('11011001')  BitMaskRealWorld=Stored Integer
  Data Type Conversion6 : DataTypeConversion  OutDataTypeStr=uint16
  Data Type Conversion7 : DataTypeConversion  OutDataTypeStr=uint16
  Shift Arithmetic2 : ArithShift  BitShiftNumber=-8
  out16b : Outport
  wires:
  low/1 -> Data Type Conversion6/1
  Bitwise Operator2/1 -> out16b/1
  high/1 -> Data Type Conversion7/1
  Data Type Conversion7/1 -> Shift Arithmetic2/1
  Shift Arithmetic2/1 -> Bitwise Operator2/2
  Data Type Conversion6/1 -> Bitwise Operator2/1

== system CubeX_LQR_2D/Read IMU/Magnetometer I2C1/Read Magnetometer Data/Turn the MSB and LSB into a signed 16-bit integer MagY ==
  low : Inport
  high : Inport  Port=2
  Bitwise Operator2 : simulink/Logic and Bit Operations/Bitwise Operator  logicop=OR  UseBitMask=off  NumInputPorts=2  BitMask=bin2dec('11011001')  BitMaskRealWorld=Stored Integer
  Data Type Conversion6 : DataTypeConversion  OutDataTypeStr=uint16
  Data Type Conversion7 : DataTypeConversion  OutDataTypeStr=uint16
  Shift Arithmetic2 : ArithShift  BitShiftNumber=-8
  out16b : Outport
  wires:
  low/1 -> Data Type Conversion6/1
  Bitwise Operator2/1 -> out16b/1
  high/1 -> Data Type Conversion7/1
  Data Type Conversion7/1 -> Shift Arithmetic2/1
  Shift Arithmetic2/1 -> Bitwise Operator2/2
  Data Type Conversion6/1 -> Bitwise Operator2/1

== system CubeX_LQR_2D/Read IMU/Magnetometer I2C1/Read Magnetometer Data/Turn the MSB and LSB into a signed 16-bit integer MagZ ==
  low : Inport
  high : Inport  Port=2
  Bitwise Operator2 : simulink/Logic and Bit Operations/Bitwise Operator  logicop=OR  UseBitMask=off  NumInputPorts=2  BitMask=bin2dec('11011001')  BitMaskRealWorld=Stored Integer
  Data Type Conversion6 : DataTypeConversion  OutDataTypeStr=uint16
  Data Type Conversion7 : DataTypeConversion  OutDataTypeStr=uint16
  Shift Arithmetic2 : ArithShift  BitShiftNumber=-8
  out16b : Outport
  wires:
  low/1 -> Data Type Conversion6/1
  Bitwise Operator2/1 -> out16b/1
  high/1 -> Data Type Conversion7/1
  Data Type Conversion7/1 -> Shift Arithmetic2/1
  Shift Arithmetic2/1 -> Bitwise Operator2/2
  Data Type Conversion6/1 -> Bitwise Operator2/1

== system CubeX_LQR_2D/Old PID and wheel velocity filter from last thesis/PID Motor 3 DONE /Subsystem/Subsystem2/Subsystem ==
  In1 : Inport
  One old speed : Inport  Port=2
  Add2 : Sum
  Gain2 : Gain  Gain=0.5
  Gain3 : Gain  Gain=0.5
  Average Speed : Outport
  One old Speed : Outport  Port=2
  wires:
  Add2/1 -> One old Speed/1, Average Speed/1  "Speed, PA1"
  One old speed/1 -> Gain2/1
  In1/1 -> Gain3/1
  Gain2/1 -> Add2/2
  Gain3/1 -> Add2/1

== system CubeX_LQR_2D/Old PID and wheel velocity filter from last thesis/PID Motor 3 DONE /Subsystem2/Subsystem1/Subsystem ==
  In1 : Inport
  One old speed : Inport  Port=2
  Add2 : Sum
  Gain2 : Gain  Gain=0.3
  Gain3 : Gain  Gain=0.7
  Average Speed : Outport
  One old Speed : Outport  Port=2
  wires:
  Add2/1 -> One old Speed/1, Average Speed/1  "Speed, PA1"
  One old speed/1 -> Gain2/1
  In1/1 -> Gain3/1
  Gain2/1 -> Add2/2
  Gain3/1 -> Add2/1

== system CubeX_LQR_2D/Read IMU/Accelometer Gyroscope I2C1/Read Accelometer and Gyroscope Data/Old gyro get data Used during SPI before/USE THIS ONE!!2 ==
  "Gyro_Zout_High " : Inport
  Gyro_Zout_Low : Inport  Port=2
  Bitwise Operator : simulink/Logic and Bit Operations/Bitwise Operator  logicop=OR  UseBitMask=off  NumInputPorts=2  BitMask=bin2dec('11011001')  BitMaskRealWorld=Stored Integer
  Data Type Conversion : DataTypeConversion  OutDataTypeStr=uint16
  Data Type Conversion1 : DataTypeConversion  OutDataTypeStr=uint16
  Shift Arithmetic : ArithShift  BitShiftNumber=-8
  Gyro_Zout : Outport
  wires:
  Gyro_Zout_Low/1 -> Data Type Conversion/1
  "Gyro_Zout_High "/1 -> Data Type Conversion1/1
  Data Type Conversion1/1 -> Shift Arithmetic/1
  Data Type Conversion/1 -> Bitwise Operator/2
  Shift Arithmetic/1 -> Bitwise Operator/1
  Bitwise Operator/1 -> Gyro_Zout/1

== system CubeX_LQR_2D/Read IMU/Accelometer Gyroscope I2C1/Read Accelometer and Gyroscope Data/Old gyro get data Used during SPI before/USE THIS ONE!!3 ==
  "Gyro_Zout_High " : Inport
  Gyro_Zout_Low : Inport  Port=2
  Bitwise Operator : simulink/Logic and Bit Operations/Bitwise Operator  logicop=OR  UseBitMask=off  NumInputPorts=2  BitMask=bin2dec('11011001')  BitMaskRealWorld=Stored Integer
  Data Type Conversion : DataTypeConversion  OutDataTypeStr=uint16
  Data Type Conversion1 : DataTypeConversion  OutDataTypeStr=uint16
  Shift Arithmetic : ArithShift  BitShiftNumber=-8
  Gyro_Zout : Outport
  wires:
  Gyro_Zout_Low/1 -> Data Type Conversion/1
  "Gyro_Zout_High "/1 -> Data Type Conversion1/1
  Data Type Conversion1/1 -> Shift Arithmetic/1
  Data Type Conversion/1 -> Bitwise Operator/2
  Shift Arithmetic/1 -> Bitwise Operator/1
  Bitwise Operator/1 -> Gyro_Zout/1

== system CubeX_LQR_2D/Read IMU/Accelometer Gyroscope I2C1/Read Accelometer and Gyroscope Data/Old gyro get data Used during SPI before/USE THIS ONE!!4 ==
  "Gyro_Zout_High " : Inport
  Gyro_Zout_Low : Inport  Port=2
  Bitwise Operator : simulink/Logic and Bit Operations/Bitwise Operator  logicop=OR  UseBitMask=off  NumInputPorts=2  BitMask=bin2dec('11011001')  BitMaskRealWorld=Stored Integer
  Data Type Conversion : DataTypeConversion  OutDataTypeStr=uint16
  Data Type Conversion1 : DataTypeConversion  OutDataTypeStr=uint16
  Shift Arithmetic : ArithShift  BitShiftNumber=-8
  Gyro_Zout : Outport
  wires:
  Gyro_Zout_Low/1 -> Data Type Conversion/1
  "Gyro_Zout_High "/1 -> Data Type Conversion1/1
  Data Type Conversion1/1 -> Shift Arithmetic/1
  Data Type Conversion/1 -> Bitwise Operator/2
  Shift Arithmetic/1 -> Bitwise Operator/1
  Bitwise Operator/1 -> Gyro_Zout/1

== system CubeX_LQR_2D/Read IMU/Accelometer Gyroscope I2C3/Read Accelometer and Gyroscope Data/Old gyro get data Used during SPI before/USE THIS ONE!!2 ==
  "Gyro_Zout_High " : Inport
  Gyro_Zout_Low : Inport  Port=2
  Bitwise Operator : simulink/Logic and Bit Operations/Bitwise Operator  logicop=OR  UseBitMask=off  NumInputPorts=2  BitMask=bin2dec('11011001')  BitMaskRealWorld=Stored Integer
  Data Type Conversion : DataTypeConversion  OutDataTypeStr=uint16
  Data Type Conversion1 : DataTypeConversion  OutDataTypeStr=uint16
  Shift Arithmetic : ArithShift  BitShiftNumber=-8
  Gyro_Zout : Outport
  wires:
  Gyro_Zout_Low/1 -> Data Type Conversion/1
  "Gyro_Zout_High "/1 -> Data Type Conversion1/1
  Data Type Conversion1/1 -> Shift Arithmetic/1
  Data Type Conversion/1 -> Bitwise Operator/2
  Shift Arithmetic/1 -> Bitwise Operator/1
  Bitwise Operator/1 -> Gyro_Zout/1

== system CubeX_LQR_2D/Read IMU/Accelometer Gyroscope I2C3/Read Accelometer and Gyroscope Data/Old gyro get data Used during SPI before/USE THIS ONE!!3 ==
  "Gyro_Zout_High " : Inport
  Gyro_Zout_Low : Inport  Port=2
  Bitwise Operator : simulink/Logic and Bit Operations/Bitwise Operator  logicop=OR  UseBitMask=off  NumInputPorts=2  BitMask=bin2dec('11011001')  BitMaskRealWorld=Stored Integer
  Data Type Conversion : DataTypeConversion  OutDataTypeStr=uint16
  Data Type Conversion1 : DataTypeConversion  OutDataTypeStr=uint16
  Shift Arithmetic : ArithShift  BitShiftNumber=-8
  Gyro_Zout : Outport
  wires:
  Gyro_Zout_Low/1 -> Data Type Conversion/1
  "Gyro_Zout_High "/1 -> Data Type Conversion1/1
  Data Type Conversion1/1 -> Shift Arithmetic/1
  Data Type Conversion/1 -> Bitwise Operator/2
  Shift Arithmetic/1 -> Bitwise Operator/1
  Bitwise Operator/1 -> Gyro_Zout/1

== system CubeX_LQR_2D/Read IMU/Accelometer Gyroscope I2C3/Read Accelometer and Gyroscope Data/Old gyro get data Used during SPI before/USE THIS ONE!!4 ==
  "Gyro_Zout_High " : Inport
  Gyro_Zout_Low : Inport  Port=2
  Bitwise Operator : simulink/Logic and Bit Operations/Bitwise Operator  logicop=OR  UseBitMask=off  NumInputPorts=2  BitMask=bin2dec('11011001')  BitMaskRealWorld=Stored Integer
  Data Type Conversion : DataTypeConversion  OutDataTypeStr=uint16
  Data Type Conversion1 : DataTypeConversion  OutDataTypeStr=uint16
  Shift Arithmetic : ArithShift  BitShiftNumber=-8
  Gyro_Zout : Outport
  wires:
  Gyro_Zout_Low/1 -> Data Type Conversion/1
  "Gyro_Zout_High "/1 -> Data Type Conversion1/1
  Data Type Conversion1/1 -> Shift Arithmetic/1
  Data Type Conversion/1 -> Bitwise Operator/2
  Shift Arithmetic/1 -> Bitwise Operator/1
  Bitwise Operator/1 -> Gyro_Zout/1

== matlab function CubeX_LQR_2D/Old PID and wheel velocity filter from last thesis/PID Motor 3 DONE /Reference calibration from buttons/Reference calibration calculation ==
  data: ref_plus input; correction_out output; ref_minus input; initial_calibration input
function correction_out = ReferenceCalibration(ref_plus,ref_minus,initial_calibration)
%#codegen

persistent correction;

delta_correction = 0.05; % NOTE: Degrees!

if isempty(correction)
    correction = initial_calibration;   % Initial calibration is estimated center of gravity offset from geometrical center, in degrees.
end

if ref_plus == 1
    correction = correction + delta_correction;
end

if ref_minus == 1
    correction = correction - delta_correction;
end

correction_out = correction;

== matlab function CubeX_LQR_2D/Read IMU/Rotation of IMU1 ==
  data: acc input; acc_out output; gyro input; gyro_out output; imu parameter
function [acc_out,gyro_out] = fcn(acc,gyro, imu)

acc_out     = imu.rot_IMU1 * single(acc);
gyro_out    = imu.rot_IMU1 * single(gyro);

== matlab function CubeX_LQR_2D/Read IMU/Magdwick Filter ==
  data: acc input single size=[1 3]; euler output single; gyro input size=[1 3]; Ts parameter
function euler = Magdwick(acc, gyro, Ts)

    persistent AHRS;
    
    if isempty(AHRS)      
       AHRS = MadgwickAHRS('SamplePeriod', Ts.IMU, 'Beta', 0.04); 
    end
    
    AHRS.UpdateIMU(gyro, acc);
    
    q = AHRS.Quaternion;
    euler = quatern2euler(quaternConj(q));

== matlab function CubeX_LQR_2D/Reference calibration from buttons/Reference calibration calculation ==
  data: ref_plus input; correction_out output; ref_minus input; inital_offset input
function correction_out = ReferenceCalibration(ref_plus,ref_minus,inital_offset)
%#codegen

persistent correction;

delta_correction = 0.02; % NOTE: Degrees!

if isempty(correction)
    correction = inital_offset;   % Initial calibration is estimated center of gravity offset from geometrical center, in degrees.
end

if ref_plus == true
    correction = correction + delta_correction;
end

if ref_minus == true
    correction = correction - delta_correction;
end

correction_out = correction;

== matlab function CubeX_LQR_2D/Read IMU/Steady State Kalman Filter ==
  data: gyro input; kf_gyro output
function kf_gyro = fcn(gyro)

persistent gyroFilter;

K = 0.1;

%init
if isempty(gyroFilter)
    gyroFilter = 0;
end

% Steady State Kalman Filter
gyroFilter = gyroFilter + K*(gyro(1) - (gyroFilter));

kf_gyro = [gyroFilter ; 0 ; 0];

== matlab function CubeX_LQR_2D/Read IMU/LP filter ==
  data: filter_acc output; acc input; gyro input; filter_gyro output
function [filter_acc,filter_gyro] = fcn(acc,gyro)

persistent f_gyro;
persistent f_acc;
persistent L_acc;
persistent L_gyro;


if isempty(f_gyro)
   f_gyro = zeros(3,1);
   f_acc  = zeros(3,1);
   Ts = 0.002;         % Sampling time
   Tf_gyro = 0.035;         % Time Constant % 0.01
   Tf_acc = 0.05;         % Time Constant % 0.05
   L_acc  = Ts/(Tf_acc + Ts);  % Filter gain
   L_gyro  = Ts/(Tf_gyro + Ts);  % Filter gain
end

% LP Filter
f_gyro = (1-L_gyro) * f_gyro + L_gyro * gyro;
f_acc  = (1-L_acc) * f_acc  + L_acc * acc;

filter_gyro = f_gyro;
filter_acc = f_acc;

== matlab function CubeX_LQR_2D/Read IMU/Moving Average filter MAF ==
  data: angle input; MAF_phi output
function MAF_phi = fcn(angle)

persistent buffer k_samples;
buffer_size = 40; %Length of filter & DEBUG 2 Seems to work
if isempty(buffer)   
    buffer = zeros(buffer_size,1);
    k_samples = 1;
end
    
buffer(k_samples,1) = angle(1);
k_samples = k_samples + 1;

if (k_samples > buffer_size)
    k_samples = 1 ;
end

MAF_phi = [mean(buffer) ; angle(2) ; angle(3) ];

== matlab function CubeX_LQR_2D/Read IMU/Lp Filter ==
  data: gyro input; filter_gyro output; Ts parameter
function filter_gyro  = fcn(gyro, Ts)

persistent f_gyro;
persistent L_gyro;


if isempty(f_gyro)
   f_gyro = zeros(3,1,'single');
   
   Tf_gyro = single(0.008);         % Time Constant % 0.04
   L_gyro  = Ts.IMU/(Tf_gyro + Ts.IMU);  % Filter gain
end

% LP Filter
f_gyro = (1-L_gyro) * f_gyro + L_gyro * gyro;
filter_gyro = single(f_gyro);

== matlab function CubeX_LQR_2D/LQR/Estimate COG offset ==
  data Ts settings: description=Sample time for LQR
  data: iref input; phi input; y output size=1; wx input; Ts parameter
function y = fcn(iref, phi, wx, Ts)
%#codegen

%Function that estimates how many the degrees the COG is offset from the
%symmetry line of the cube. 


persistent phi_offs k_min k iref_mean 

if(isempty(phi_offs))
   phi_offs = zeros(1,1,'single');
   Tmin = single(0.4);                 %Wait at least this long before incrementing
   k_min = single(round(Tmin/Ts.controller)); 
   k = zeros(1,1,'single');  
   iref_mean = zeros(1,1,'single'); 
end

%Tuning factor, normalized to the sampling speed of the algoritmh so phi 
%is increased by the same angular rate [rad/s] no matter what Ts is
%chosen
c = -0.19*Ts.controller;
%c=0;

%Wait k_min sample in a stable area before deciding to to anything 
if( abs(wx) < 0.03 && abs(phi) < deg2rad(2) ) 
    k = k + 1; 
    iref_mean = iref_mean + iref; 
    
    if(k > k_min)        
       iref_mean = iref_mean/(k_min+1); 
       phi_offs = phi_offs + c*iref_mean;  
       k = zeros(1,1,'single'); 
       iref_mean = zeros(1,1,'single'); 
    end
    
else
    iref_mean = zeros(1,1,'single');  
    k = zeros(1,1,'single'); 
end

if abs(phi_offs) > 0.8726 % 50 degress
    phi_offs = zeros(1,1,'single');
end
y = phi_offs;

== matlab function CubeX_LQR_2D/Read IMU/Accelometer Gyroscope I2C3/Read Accelometer and Gyroscope Data/Old gyro get data Used during SPI before/Take away Sensor fail reading ==
  data: y output; new input; old input
function y = fcn(new, old)
%#codegen
if(new > -257 && new < -200)
   y = old;
else
    y = new;
end

== matlab function CubeX_LQR_2D/Read IMU/Accelometer Gyroscope I2C3/Read Accelometer and Gyroscope Data/Old gyro get data Used during SPI before/Take away Sensor fail reading if two bad in raw ==
  data: y output; new input; old input
function y = fcn(new, old)
%#codegen
if(new > -257 && new < -200)
   y = old;
else
    y = new;
end

== matlab function CubeX_LQR_2D/Read IMU/Accelometer Gyroscope I2C3/Read Accelometer and Gyroscope Data/Old gyro get data Used during SPI before/Take away Sensor fail reading if two bad in raw1 ==
  data: y output; new input; old input
function y = fcn(new, old)
%#codegen
if(new > -257 && new < -200)
   y = old;
else
    y = new;
end

== matlab function CubeX_LQR_2D/Read IMU/Accelometer Gyroscope I2C3/Read Accelometer and Gyroscope Data/Old gyro get data Used during SPI before/Take away Sensor fail reading if two bad in raw2 ==
  data: y output; new input; old input
function y = fcn(new, old)
%#codegen
if(new > -257 && new < -200)
   y = old;
else
    y = new;
end

== matlab function CubeX_LQR_2D/READ ACC AND GYRO WITH SPI/Take away Sensor fail reading ==
  data: y output; new input; old input
function y = fcn(new, old)
%#codegen
if(new > -257 && new < -200)
   y = old;
else
    y = new;
end

== matlab function CubeX_LQR_2D/READ ACC AND GYRO WITH SPI/Take away Sensor fail reading if two bad in raw ==
  data: y output; new input; old input
function y = fcn(new, old)
%#codegen
if(new > -257 && new < -200)
   y = old;
else
    y = new;
end

== matlab function CubeX_LQR_2D/Read IMU/Accelometer Gyroscope I2C3/Read Accelometer and Gyroscope Data/Old gyro get data Used during SPI before/Take away Sensor fail reading1 ==
  data: y output; new input; old input
function y = fcn(new, old)
%#codegen
if(new > -257 && new < -200)
   y = old;
else
    y = new;
end

== matlab function CubeX_LQR_2D/Read IMU/Accelometer Gyroscope I2C3/Read Accelometer and Gyroscope Data/Old gyro get data Used during SPI before/Take away Sensor fail reading2 ==
  data: y output; new input; old input
function y = fcn(new, old)
%#codegen
if(new > -257 && new < -200)
   y = old;
else
    y = new;
end

== matlab function CubeX_LQR_2D/Read IMU/Rotation of IMU3 ==
  data: acc input; acc_out output; gyro input; gyro_out output; imu parameter
function [acc_out,gyro_out] = fcn(acc,gyro, imu)

acc_out     = imu.rot_IMU3 * single(acc);
gyro_out    = imu.rot_IMU3 * single(gyro);
